simulink model "SMC_dc_dc_Conv"  (R2022b)
settings: Solver=ode23s  StartTime=0.0  StopTime=5  MaxStep=1e-4  RelTol=1e-3
libraries: spsSeriesRLCBranchLib x3, spsCurrentMeasurementLib x1, spsDCVoltageSourceLib x1, spsDiodeLib x1, spsIGBTDiodeLib x1, spsVoltageMeasurementLib x1, spspowerguiLib x1
settings Model: Creator=User  LastModifiedBy=Lenovo
settings OptimizationCC: ReuseModelBlockBuffer=on

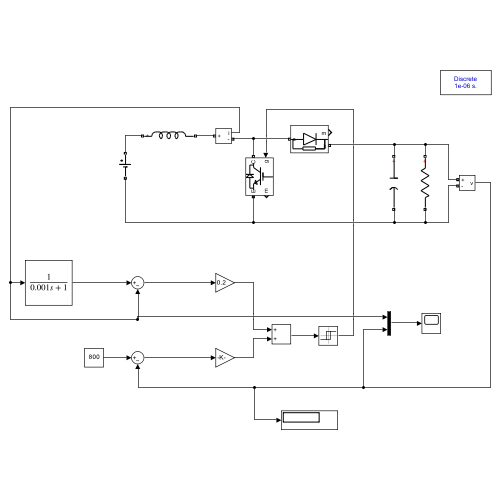
[thumbnail: Simulink's stored preview of the top-level diagram]
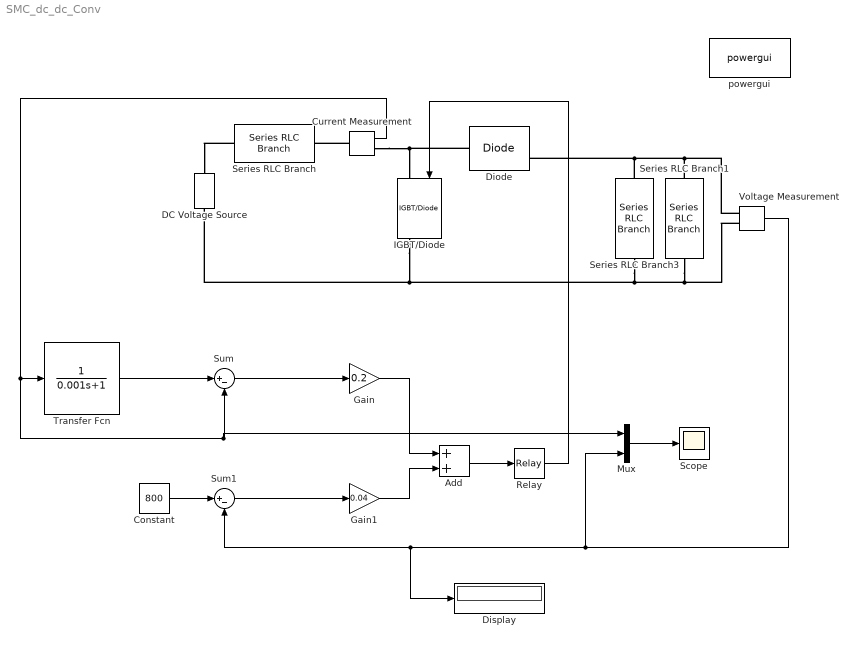
== system SMC_dc_dc_Conv ==
  Add : Sum
  Constant : Constant  Value=800
  Current Measurement : spsCurrentMeasurementLib/Current Measurement  PhasorSimulation=off  OutputType=Complex  PSBequivalent=0
  DC Voltage Source : spsDCVoltageSourceLib/DC Voltage Source  Amplitude=100  Measurements=None
  Diode : spsDiodeLib/Diode  Ron=0.001  Lon=0  Vf=0.8  IC=0  UseSnubber=0  Rs=500  Cs=250e-9  Measurements=on
  Display : Display
  Gain : Gain  Gain=0.2
  Gain1 : Gain  Gain=0.04
  IGBT/Diode : spsIGBTDiodeLib/IGBT//Diode  Ron=1e-3  Rs=1e5  Cs=inf  Measurements=on
  Mux : Mux  Inputs=2
  Relay : Relay  OnSwitchValue=0.1  OffSwitchValue=-0.1
  Scope : Scope
  Series RLC Branch : spsSeriesRLCBranchLib/Series RLC Branch  LConnTagsString=__new0  RConnTagsString=__new0  BranchType=L  Resistance=1  Inductance=1e-3  SetiL0=off  InitialCurrent=0  Capacitance=1e-6  Setx0=off  InitialVoltage=0  Measurements=None
  Series RLC Branch1 : spsSeriesRLCBranchLib/Series RLC Branch  LConnTagsString=__new0  RConnTagsString=__new0  BranchType=R  Resistance=100  Inductance=1e-3  SetiL0=off  InitialCurrent=0  Capacitance=1e-6  Setx0=off  InitialVoltage=0  Measurements=None
  Series RLC Branch3 : spsSeriesRLCBranchLib/Series RLC Branch  LConnTagsString=__new0  RConnTagsString=__new0  BranchType=C  Resistance=1  Inductance=1e-3  SetiL0=off  InitialCurrent=0  Capacitance=100e-6  Setx0=off  InitialVoltage=0  Measurements=None
  Sum : Sum  Inputs=|+-
  Sum1 : Sum  Inputs=|+-
  Transfer Fcn : TransferFcn  Denominator=[0.001 1]
  Voltage Measurement : spsVoltageMeasurementLib/Voltage Measurement  PhasorSimulation=off  OutputType=Complex  PSBequivalent=0
  powergui : spspowerguiLib/powergui  Priority=1  SimulationMode=Discrete  SampleTime=1e-6  frequency=60  Iterations=50  frequencyindice=0  Pbase=100e6  ErrMax=1e-4  UnitsV=kV  UnitsW=MW  buscounter=0  FunctionMessages=off  echomessages=off  EnableUseOfTLC=off  CurrentSourceSwitches=off  DisableSnubberDevices=off  DisableRonSwitches=off  DisableVfSwitches=off  DisplayEquations=off  AutomaticDiscreteSolvers=off  SolverType=Tustin/Backward Euler (TBE)  Interpol=off  ExternalGateDelay=off  methode=off  Ts=100  x0status=blocks  SPID=on  SwTol=0  HookPort=off  NonlinearTolerance=1e-4  nMaxIteration=100  ContinueOnMaxIteration=off  RestoreLinks=warning  ResistiveCurrentMeasurement=off  Frange=[0:2:500]  Ylog=off  Xlog=on  ShowGrid=off  save=off  variable=ZData  structure=0  ZoomFFT=off  StartTime=0.0  cycles=1  DisplayStyle=1  fundamental=60  FreqAxis=off  MaxFrequency=1000  frequencyindicesteady=1  RmsSteady=1  display=off
  wires:
  Add/1 -> Relay/1
  Gain/1 -> Add/1
  Gain1/1 -> Add/2
  Voltage Measurement/1 -> Mux/2, Display/1, Sum1/2
  Sum1/1 -> Gain1/1
  Relay/1 -> IGBT/Diode/1
  Constant/1 -> Sum1/1
  Sum/1 -> Gain/1
  Transfer Fcn/1 -> Sum/1
  Current Measurement/1 -> Mux/1, Sum/2, Transfer Fcn/1
  Mux/1 -> Scope/1
  connections:
  Diode/LConn1 -- Current Measurement/RConn1 -- IGBT/Diode/LConn1
  Series RLC Branch/LConn1 -- DC Voltage Source/RConn1
  Series RLC Branch1/LConn1 -- Series RLC Branch3/LConn1 -- Diode/RConn1 -- Voltage Measurement/LConn1
  Current Measurement/LConn1 -- Series RLC Branch/RConn1
  Series RLC Branch1/RConn1 -- Voltage Measurement/LConn2 -- Series RLC Branch3/RConn1 -- IGBT/Diode/RConn1 -- DC Voltage Source/LConn1
